simulink model "PIDtestP2"  (R2016b)
settings: Solver=FixedStepAuto  StartTime=0.0  StopTime=15  MaxStep=0.1  RelTol=1e-3  EnableMultiTasking=on
values from neighbouring files (symbols this model uses):
  CV01 = 100    [PIDValveTest.m]    (also in PIDtestP2m.m; loggingTest.m)
  CV01t = 0.5    [PIDValveTest.m]    (also in PIDtestP2m.m; gatherData.m = 5)
  Kd = ZNTd(i)    [PIDValveTest.m]    (also in PIDtestP2m.m)
  Ki = ZNTi(i)    [PIDValveTest.m]    (also in PIDtestP2m.m)
  Kn = 0    [PIDValveTest.m]    (also in PIDtestP2m.m = 100)
  Kp = ZNKp(i)    [PIDValveTest.m]    (also in PIDtestP2m.m = 500)
  setpoint = 1    [PIDValveTest.m]
  simstop = 60*1    (= 60)    [PIDValveTest.m]    (also in PIDtestP2m.m = 30; gatherData.m = (numel(WPtime))*10+CV01t)
libraries: xpcnilib x2, slrtlib x2, simulink x1
settings Model: ModifiedByFormat=The MathWorks Inc.  Creator=The MathWorks, Inc.  LastModifiedBy=The MathWorks Inc.
settings SolverCC: EnableConcurrentExecution=on
settings DataIOCC: LimitDataPoints=on  SaveFormat=Array
settings OptimizationCC: BlockReduction=off  DefaultParameterBehavior=Inlined  OptimizeBlockIOStorage=off  BufferReuse=off  GlobalBufferReuse=off  ExpressionFolding=off  ExpressionDepthLimit=2147483647  LocalBlockOutputs=off  LifeSpan=inf
settings DebuggingCC: UnderspecifiedInitializationDetection=Classic  MergeDetectMultiDrivingBlocksExec=none  SolverPrmCheckMsg=warning  FcnCallInpInsideContextMsg=warning  AllowSymbolicDim=off  StateNameClashWarn=warning  SFUnexpectedBacktrackingDiag=warning  SFNoUnconditionalDefaultTransitionDiag=warning  SFExecutionAtInitializationDiag=none
settings HardwareCC: ProdBitPerPointer=32  ProdBitPerSizeT=32  ProdBitPerPtrDiffT=32  ProdLargestAtomicFloat=None  ProdWordSize=32  ProdLongLongMode=on  ProdHWDeviceType=Generic->32-bit x86 compatible
settings ModelReferenceCC: ModelReferenceNumInstancesAllowed=Single  ModelReferenceMinAlgLoopOccurrences=on  PropagateSignalLabelsOutOfModel=off
settings RTWCC: SystemTargetFile=slrt.tlc  TemplateMakefile=slrt_default_tmf  Description=Simulink Real-Time  RTWVerbose=off
settings ConfigComp: CovMetricSettings=dw  CovHtmlReporting=on  CovSaveCumulativeToWorkspaceVar=on  CovSaveSingleToWorkspaceVar=on  CovExternalEMLEnable=off  CovSFcnEnable=off

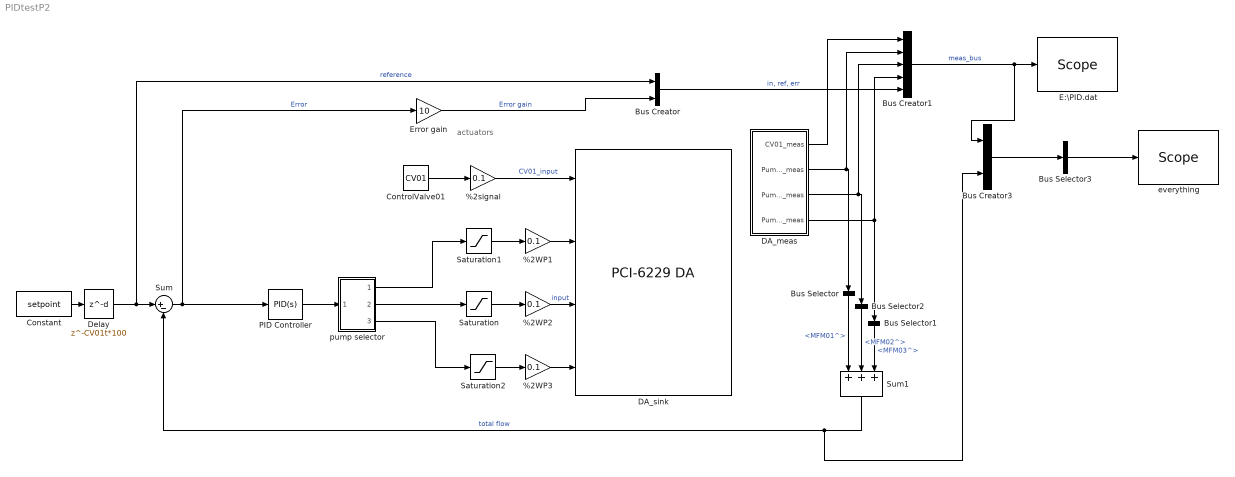
== system PIDtestP2 ==
  note: actuators
  %2WP1 : Gain  Gain=0.1
  %2WP2 : Gain  Gain=0.1
  %2WP3 : Gain  Gain=0.1
  %2signal : Gain  Gain=0.1
  Bus Creator : BusCreator  Inputs=3
  Bus Creator1 : BusCreator  Inputs=5
  Bus Creator3 : BusCreator  Inputs=2
  Bus Selector : BusSelector  OutputSignals=MFM01^
  Bus Selector1 : BusSelector  OutputSignals=MFM03^
  Bus Selector2 : BusSelector  OutputSignals=MFM02^
  Bus Selector3 : BusSelector  OutputSignals=meas_bus.Pump1.MFM01^,meas_bus.Pump2.MFM02^,meas_bus.Pump3.MFM03^,total flow,meas_bus.in; ref; err  OutputAsBus=on
  Constant : Constant  Value=setpoint
  ControlValve01 : Constant  Value=CV01
  DA_meas : Subsystem
  DA_sink : xpcnilib/D//A/M Series/PCI-6229 DA  channel=[4 1 2 3]  reset=[1]  initValue=[0]  sampletime=0.01  slot=-1
  Delay : Delay  DelayLength=CV01t*100
  E:\PID.dat : slrtlib/Displays and Logging/Scope   scopeno=20  scopetype=File  autostart=on  viewmode=Graphical sliding  formatstr='%15.6f'  grid=on  ylimits=[0,0]  nosamples=100*simstop  noprepostsamples=0  interleave=1  triggermode=FreeRun  triggersignal=1  trigsignalfromport=off  triggerlevel=0.0  triggerslope=Either  triggerscope=1  triggersample=0  filename=E:\PID.dat  mode=Lazy  writesize=512  autorestart=off  dynamicfilemode=off  maxwritefilesize=512*1024^2
  Error gain : Gain  Gain=10
  PID Controller : simulink/Continuous/PID Controller  Controller=PID  TimeDomain=Continuous-time  SampleTime=-1  IntegratorMethod=Forward Euler  FilterMethod=Forward Euler  Form=Parallel  UseFilter=on  ControllerParametersSource=internal  P=Kp  I=Ki  D=Kd  N=Kn  InitialConditionSource=internal  InitialConditionForIntegrator=0  InitialConditionForFilter=0  ExternalReset=none  LimitOutput=off  UpperSaturationLimit=inf  LowerSaturationLimit=-inf  LinearizeAsGain=on  AntiWindupMode=none  Kb=1  TrackingMode=off  Kt=1  PParamMin=[]  PParamMax=[]  IParamMin=[]  IParamMax=[]  DParamMin=[]  DParamMax=[]  NParamMin=[]  NParamMax=[]  KbParamMin=[]  KbParamMax=[]  KtParamMin=[]  KtParamMax=[]  POutMin=[]  POutMax=[]  IOutMin=[]  IOutMax=[]  DOutMin=[]  DOutMax=[]  NOutMin=[]  NOutMax=[]  KbOutMin=[]  KbOutMax=[]  KtOutMin=[]  KtOutMax=[]  IntegratorOutMin=[]  IntegratorOutMax=[]  FilterOutMin=[]  FilterOutMax=[]  SumOutMin=[]  SumOutMax=[]  SumI1OutMin=[]  SumI1OutMax=[]  SumI2OutMin=[]  SumI2OutMax=[]  SumI3OutMin=[]  SumI3OutMax=[]  SumDOutMin=[]  SumDOutMax=[]  SaturationOutMin=[]  SaturationOutMax=[]  IntegratorContinuousStateAttributes=''  IntegratorStateMustResolveToSignalObject=off  IntegratorRTWStateStorageClass=Auto  FilterContinuousStateAttributes=''  FilterStateMustResolveToSignalObject=off  FilterRTWStateStorageClass=Auto  DifferentiatorICPrevScaledInput=0  DifferentiatorOutMin=[]  DifferentiatorOutMax=[]
  Saturation : Saturate  UpperLimit=80  LowerLimit=0
  Saturation1 : Saturate  UpperLimit=80  LowerLimit=0
  Saturation2 : Saturate  UpperLimit=80  LowerLimit=0
  Sum : Sum  Inputs=|+-
  Sum1 : Sum  Inputs=+++
  everything : slrtlib/Displays and Logging/Scope   scopeno=10  scopetype=Target  autostart=on  viewmode=Graphical sliding  formatstr='%15.6f'  grid=on  ylimits=[-30,30]  nosamples=100*simstop  noprepostsamples=0  interleave=1  triggermode=FreeRun  triggersignal=1  trigsignalfromport=off  triggerlevel=0.0  triggerslope=Either  triggerscope=1  triggersample=0  filename=E:\unused1.dat  mode=Lazy  writesize=512  autorestart=off  dynamicfilemode=off  maxwritefilesize=512*1024^2
  pump selector : Subsystem
  wires:
  pump selector/3(Out3) -> Saturation2/1
  pump selector/1(Out1) -> Saturation1/1
  ControlValve01/1 -> %2signal/1
  %2signal/1 -> DA_sink/1  "CV01_input"
  %2WP1/1 -> DA_sink/2
  %2WP3/1 -> DA_sink/4
  DA_meas/4(Pump3_meas) -> Bus Creator1/4, Bus Selector1/1
  DA_meas/2(Pump1_meas) -> Bus Creator1/2, Bus Selector/1
  DA_meas/3(Pump2_meas) -> Bus Creator1/3, Bus Selector2/1
  Bus Creator1/1 -> Bus Creator3/1, E:\PID.dat/1  "meas_bus"
  Bus Selector/1 -> Sum1/1  "<MFM01^>"
  Bus Selector2/1 -> Sum1/2  "<MFM02^>"
  Bus Selector1/1 -> Sum1/3  "<MFM03^>"
  Sum1/1 -> Sum/2, Bus Creator3/2  "total flow"
  Constant/1 -> Delay/1
  %2WP2/1 -> DA_sink/3  "input"
  Delay/1 -> Bus Creator/1, Sum/1  "reference"
  Saturation/1 -> %2WP2/1
  Bus Creator3/1 -> Bus Selector3/1
  Sum/1 -> PID Controller/1, Error gain/1  "Error"
  Error gain/1 -> Bus Creator/3  "Error gain"
  DA_meas/1(CV01_meas) -> Bus Creator1/1
  Bus Selector3/1 -> everything/1
  Bus Creator/1 -> Bus Creator1/5  "in, ref, err"
  Saturation1/1 -> %2WP1/1
  Saturation2/1 -> %2WP3/1
  pump selector/2(Out2) -> Saturation/1
  PID Controller/1 -> pump selector/1(In1)

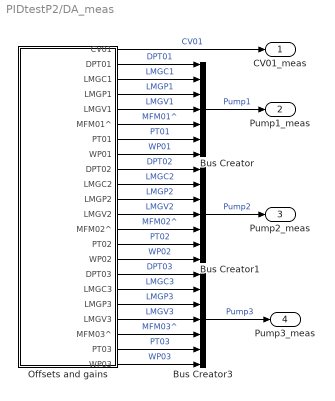
== system PIDtestP2/DA_meas ==
  Bus Creator : BusCreator  Inputs=7
  Bus Creator1 : BusCreator  Inputs=7
  Bus Creator3 : BusCreator  Inputs=7
  Offsets and gains : Subsystem
  CV01_meas : Outport
  Pump1_meas : Outport  Port=2
  Pump2_meas : Outport  Port=3
  Pump3_meas : Outport  Port=4
  wires:
  Bus Creator/1 -> Pump1_meas/1  "Pump1"
  Bus Creator1/1 -> Pump2_meas/1  "Pump2"
  Bus Creator3/1 -> Pump3_meas/1  "Pump3"
  Offsets and gains/8(WP01) -> Bus Creator/7  "WP01"
  Offsets and gains/9(DPT02) -> Bus Creator1/1  "DPT02"
  Offsets and gains/4(LMGP1) -> Bus Creator/3  "LMGP1"
  Offsets and gains/2(DPT01) -> Bus Creator/1  "DPT01"
  Offsets and gains/1(CV01) -> CV01_meas/1  "CV01"
  Offsets and gains/11(LMGP2) -> Bus Creator1/3  "LMGP2"
  Offsets and gains/15(WP02) -> Bus Creator1/7  "WP02"
  Offsets and gains/18(LMGP3) -> Bus Creator3/3  "LMGP3"
  Offsets and gains/22(WP03) -> Bus Creator3/7  "WP03"
  Offsets and gains/6(MFM01^) -> Bus Creator/5  "MFM01^"
  Offsets and gains/20(MFM03^) -> Bus Creator3/5  "MFM03^"
  Offsets and gains/10(LMGC2) -> Bus Creator1/2  "LMGC2"
  Offsets and gains/12(LMGV2) -> Bus Creator1/4  "LMGV2"
  Offsets and gains/13(MFM02^) -> Bus Creator1/5  "MFM02^"
  Offsets and gains/14(PT02) -> Bus Creator1/6  "PT02"
  Offsets and gains/19(LMGV3) -> Bus Creator3/4  "LMGV3"
  Offsets and gains/21(PT03) -> Bus Creator3/6  "PT03"
  Offsets and gains/16(DPT03) -> Bus Creator3/1  "DPT03"
  Offsets and gains/17(LMGC3) -> Bus Creator3/2  "LMGC3"
  Offsets and gains/3(LMGC1) -> Bus Creator/2  "LMGC1"
  Offsets and gains/5(LMGV1) -> Bus Creator/4  "LMGV1"
  Offsets and gains/7(PT01) -> Bus Creator/6  "PT01"

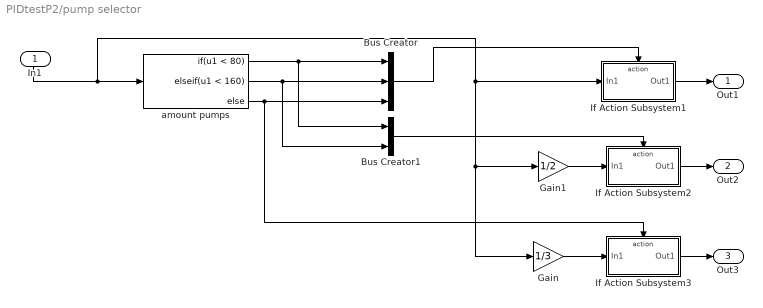
== system PIDtestP2/pump selector ==
  In1 : Inport
  Bus Creator : BusCreator  Inputs=3
  Bus Creator1 : BusCreator  Inputs=2
  Gain : Gain  Gain=1/3
  Gain1 : Gain  Gain=1/2
  If Action Subsystem1 : Subsystem  TreatAsAtomicUnit=on
  If Action Subsystem2 : Subsystem  TreatAsAtomicUnit=on
  If Action Subsystem3 : Subsystem  TreatAsAtomicUnit=on
  amount pumps : If  IfExpression=u1 < 80  ElseIfExpressions=u1 < 160
  Out1 : Outport
  Out2 : Outport  Port=2
  Out3 : Outport  Port=3
  wires:
  In1/1 -> If Action Subsystem1/1(In1), Gain1/1, Gain/1, amount pumps/1
  amount pumps/1 -> Bus Creator1/1, Bus Creator/1
  amount pumps/2 -> Bus Creator1/2, Bus Creator/2
  amount pumps/3 -> If Action Subsystem3/Action, Bus Creator/3
  Bus Creator/1 -> If Action Subsystem1/Action
  Bus Creator1/1 -> If Action Subsystem2/Action
  If Action Subsystem1/1(Out1) -> Out1/1
  If Action Subsystem2/1(Out1) -> Out2/1
  If Action Subsystem3/1(Out1) -> Out3/1
  Gain/1 -> If Action Subsystem3/1(In1)
  Gain1/1 -> If Action Subsystem2/1(In1)

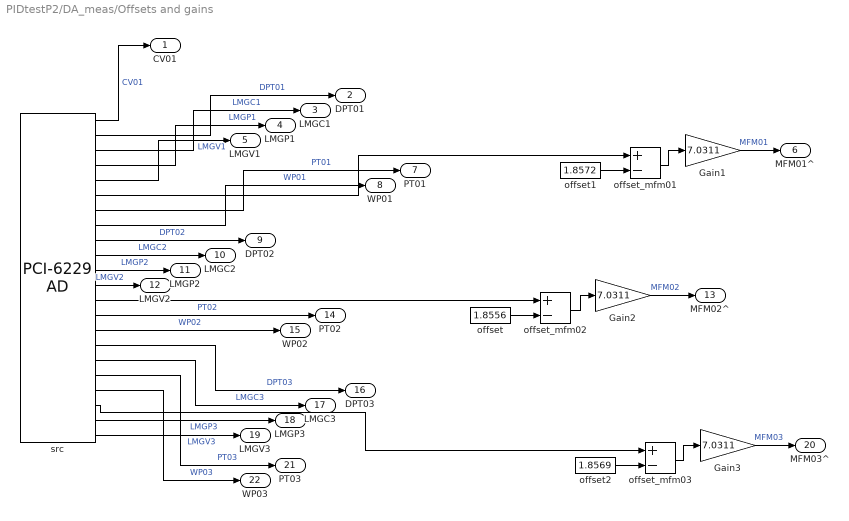
== system PIDtestP2/DA_meas/Offsets and gains ==
  Gain1 : Gain  Gain=7.0311
  Gain2 : Gain  Gain=7.0311
  Gain3 : Gain  Gain=7.0311
  offset : Constant  Value=1.8556
  offset1 : Constant  Value=1.8572
  offset2 : Constant  Value=1.8569
  offset_mfm01 : Sum  Inputs=+-
  offset_mfm02 : Sum  Inputs=+-
  offset_mfm03 : Sum  Inputs=+-
  src : xpcnilib/A//D/M Series/PCI-6229 AD  channel=[4 17 5 11 8 21 24 1 18 6 12 9 22 25 2 19 7 13 10 23 26 3]  range=[10]  coupling=[0]  scantime=5e-6  sampletime=0.01  slot=-1
  CV01 : Outport
  DPT01 : Outport  Port=2
  LMGC1 : Outport  Port=3
  LMGP1 : Outport  Port=4
  LMGV1 : Outport  Port=5
  MFM01^ : Outport  Port=6
  PT01 : Outport  Port=7
  WP01 : Outport  Port=8
  DPT02 : Outport  Port=9
  LMGC2 : Outport  Port=10
  LMGP2 : Outport  Port=11
  LMGV2 : Outport  Port=12
  MFM02^ : Outport  Port=13
  PT02 : Outport  Port=14
  WP02 : Outport  Port=15
  DPT03 : Outport  Port=16
  LMGC3 : Outport  Port=17
  LMGP3 : Outport  Port=18
  LMGV3 : Outport  Port=19
  MFM03^ : Outport  Port=20
  PT03 : Outport  Port=21
  WP03 : Outport  Port=22
  wires:
  src/18 -> LMGP3/1  "LMGP3"
  src/19 -> LMGV3/1  "LMGV3"
  src/22 -> WP03/1  "WP03"
  src/21 -> PT03/1  "PT03"
  src/10 -> LMGC2/1  "LMGC2"
  src/12 -> LMGV2/1  "LMGV2"
  src/15 -> WP02/1  "WP02"
  src/3 -> LMGC1/1  "LMGC1"
  src/9 -> DPT02/1  "DPT02"
  src/11 -> LMGP2/1  "LMGP2"
  src/14 -> PT02/1  "PT02"
  src/16 -> DPT03/1  "DPT03"
  src/17 -> LMGC3/1  "LMGC3"
  src/2 -> DPT01/1  "DPT01"
  src/1 -> CV01/1  "CV01"
  Gain3/1 -> MFM03^/1  "MFM03"
  offset1/1 -> offset_mfm01/2
  src/4 -> LMGP1/1  "LMGP1"
  src/5 -> LMGV1/1  "LMGV1"
  src/7 -> PT01/1  "PT01"
  src/8 -> WP01/1  "WP01"
  offset2/1 -> offset_mfm03/2
  offset_mfm03/1 -> Gain3/1
  offset_mfm01/1 -> Gain1/1
  src/6 -> offset_mfm01/1
  src/20 -> offset_mfm03/1
  src/13 -> offset_mfm02/1
  offset_mfm02/1 -> Gain2/1
  offset/1 -> offset_mfm02/2
  Gain2/1 -> MFM02^/1  "MFM02"
  Gain1/1 -> MFM01^/1  "MFM01"

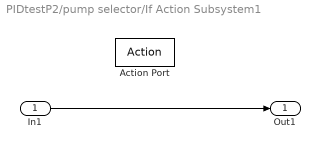
== system PIDtestP2/pump selector/If Action Subsystem1 ==
  In1 : Inport
  Action Port : ActionPort
  Out1 : Outport
  wires:
  In1/1 -> Out1/1

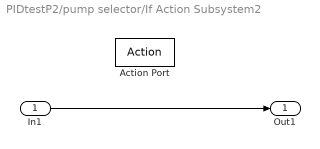
== system PIDtestP2/pump selector/If Action Subsystem2 ==
  In1 : Inport
  Action Port : ActionPort
  Out1 : Outport
  wires:
  In1/1 -> Out1/1

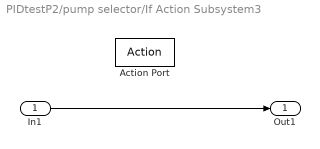
== system PIDtestP2/pump selector/If Action Subsystem3 ==
  In1 : Inport
  Action Port : ActionPort  ActionType=else
  Out1 : Outport
  wires:
  In1/1 -> Out1/1
